simulink model "sampleModel2090"  (R2023a)
settings: Solver=VariableStepAuto  StartTime=0.0  StopTime=10.0  RelTol=1e-3
libraries: hdlsllib x8
settings Model: Creator=user1  LastModifiedBy=user1

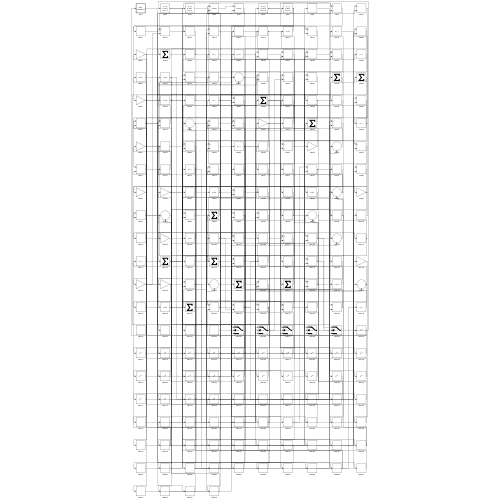
[thumbnail: Simulink's stored preview of the top-level diagram]
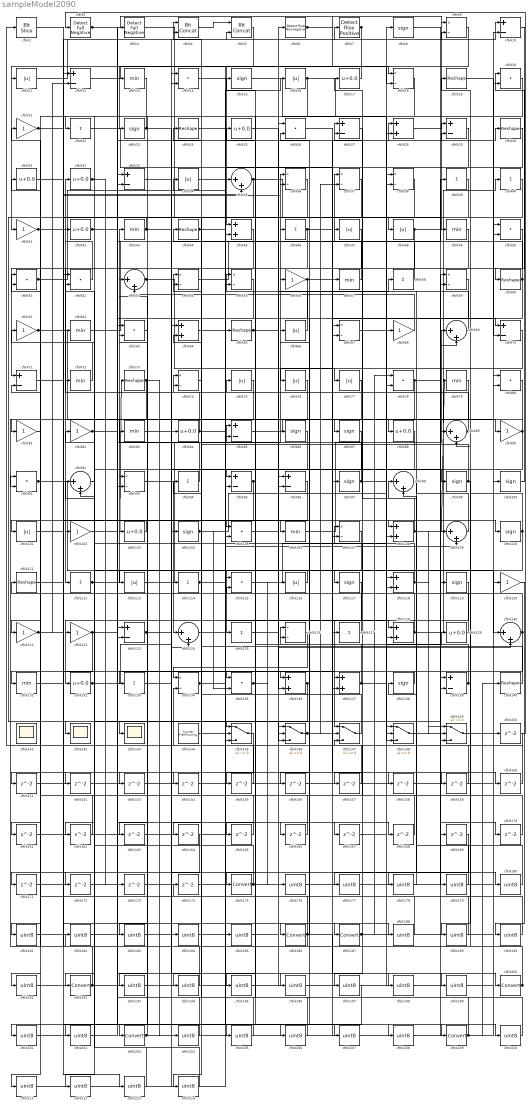
== system sampleModel2090 ==
  cfblk1 : hdlsllib/Logic and Bit Operations/Bit Slice  lidx=7  ridx=0
  cfblk{10,12,27,29,33,70..71,85,95..96,123,139} (12 alike) : Sum  Inputs=+-
  cfblk{8,15,23,86..87,97,99..100,104,110,117,119,138} (13 alike) : Signum
  cfblk{11,16,34,47..48,66,75..77,101,113,116} (12 alike) : Abs  SaturateOnIntegerOverflow=off
  cfblk{21,41,56,61,68,81..82,90,102,120..122} (12 alike) : Gain
  cfblk{17,25,31..32,42,84,88,103,129,132} (10 alike) : Bias  Bias=0.0  SaturateOnIntegerOverflow=off
  cfblk{14,20,26,50..52,63,78,80,91,105,115,135} (13 alike) : DotProduct  OutDataTypeStr=Inherit: Inherit via internal rule
  cfblk{13,43,49,57,62,72,79,83,106,131} (10 alike) : MinMax
  cfblk{9,18,36..38,54..55,59,67,74,93,107,126,134} (14 alike) : Product  Inputs=*/  RndMeth=Zero  SaturateOnIntegerOverflow=on
  cfblk{28,45,64,108,118,128,136..137} (8 alike) : Sum
  cfblk{35,53,69,89,92,98,109,124,130} (9 alike) : Sum  Inputs=|++
  cfblk{19,24,30,44,60,65,73,111,140} (9 alike) : Reshape
  cfblk{22,39..40,46,58,94,112,114,125,127,133} (11 alike) : Sum  Inputs=+
  cfblk141 : Scope
      settings: Floating=on
  cfblk142 : Scope
  cfblk143 : Scope
  cfblk144 : hdlsllib/Sources/Counter Free-Running  NumBits=16  tsamp=-1
  cfblk{145..149} (5 alike) : Switch  SaturateOnIntegerOverflow=off  InputSameDT=off
  cfblk{150..174} (25 alike) : Delay  SampleTime=1
  cfblk{175,186..187,192,200,203,209} (7 alike) : DataTypeConversion  SaturateOnIntegerOverflow=off  RndMeth=Floor
  cfblk{176..185,188..191,193..199,201..202,204..208,210..214} (33 alike) : DataTypeConversion  OutDataTypeStr=uint8  SaturateOnIntegerOverflow=off  RndMeth=Floor
  cfblk2 : hdlsllib/Logic and Bit Operations/Detect Fall Negative  vinit=0  OutDataTypeStr=boolean
  cfblk3 : hdlsllib/Logic and Bit Operations/Detect Fall Negative  vinit=0  OutDataTypeStr=boolean
  cfblk4 : hdlsllib/Logic and Bit Operations/Bit Concat  numInputs=2
  cfblk5 : hdlsllib/Logic and Bit Operations/Bit Concat  numInputs=2
  cfblk6 : hdlsllib/Logic and Bit Operations/Detect Rise Nonnegative  vinit=0  OutDataTypeStr=boolean
  cfblk7 : hdlsllib/Logic and Bit Operations/Detect Rise Positive  vinit=0  OutDataTypeStr=boolean
  wires:
  cfblk94/1 -> cfblk43/1
  cfblk86/1 -> cfblk192/1
  cfblk107/1 -> cfblk125/1
  cfblk128/1 -> cfblk40/1, cfblk54/2
  cfblk43/1 -> cfblk142/1, cfblk105/1
  cfblk52/1 -> cfblk32/1
  cfblk112/1 -> cfblk73/1, cfblk46/1, cfblk168/1
  cfblk44/1 -> cfblk166/1, cfblk167/1
  cfblk3/1 -> cfblk136/1
  cfblk2/1 -> cfblk49/1, cfblk148/3
  cfblk55/1 -> cfblk123/2
  cfblk42/1 -> cfblk3/1, cfblk137/2
  cfblk126/1 -> cfblk134/1
  cfblk45/1 -> cfblk112/1
  cfblk7/1 -> cfblk45/1, cfblk23/1
  cfblk77/1 -> cfblk103/1
  cfblk133/1 -> cfblk84/1
  cfblk57/1 -> cfblk37/1
  cfblk64/1 -> cfblk187/1
  cfblk31/1 -> cfblk106/1
  cfblk66/1 -> cfblk36/1
  cfblk18/1 -> cfblk95/1
  cfblk73/1 -> cfblk93/2, cfblk184/1
  cfblk85/1 -> cfblk90/1
  cfblk10/1 -> cfblk60/1
  cfblk28/1 -> cfblk29/1
  cfblk27/1 -> cfblk87/1
  cfblk117/1 -> cfblk147/1
  cfblk106/1 -> cfblk69/1
  cfblk122/1 -> cfblk85/1, cfblk131/1
  cfblk9/1 -> cfblk41/1
  cfblk37/1 -> cfblk81/1
  cfblk119/1 -> cfblk132/1
  cfblk90/1 -> cfblk83/1, cfblk156/1
  cfblk89/1 -> cfblk25/1, cfblk4/2
  cfblk108/1 -> cfblk79/1, cfblk17/1, cfblk149/1
  cfblk115/1 -> cfblk8/1
  cfblk65/1 -> cfblk145/1, cfblk58/1, cfblk130/2, cfblk165/1
  cfblk113/1 -> cfblk56/1
  cfblk48/1 -> cfblk119/1, cfblk205/1
  cfblk8/1 -> cfblk139/1
  cfblk4/1 -> cfblk5/1
  cfblk139/1 -> cfblk126/1, cfblk15/1
  cfblk5/1 -> cfblk85/2
  cfblk51/1 -> cfblk34/1, cfblk188/1
  cfblk33/1 -> cfblk200/1
  cfblk125/1 -> cfblk27/1
  cfblk35/1 -> cfblk69/2, cfblk191/1
  cfblk62/1 -> cfblk39/1
  cfblk22/1 -> cfblk97/1
  cfblk69/1 -> cfblk27/2
  cfblk67/1 -> cfblk68/1
  cfblk146/1 -> cfblk57/1, cfblk37/2
  cfblk47/1 -> cfblk71/1
  cfblk50/1 -> cfblk175/1
  cfblk56/1 -> cfblk70/1, cfblk30/1, cfblk133/1
  cfblk72/1 -> cfblk21/1
  cfblk88/1 -> cfblk117/1
  cfblk93/1 -> cfblk124/1
  cfblk14/1 -> cfblk209/1
  cfblk97/1 -> cfblk148/1, cfblk54/1
  cfblk135/1 -> cfblk116/1, cfblk176/1
  cfblk63/1 -> cfblk203/1
  cfblk58/1 -> cfblk44/1
  cfblk137/1 -> cfblk75/1, cfblk129/1
  cfblk24/1 -> cfblk128/1
  cfblk68/1 -> cfblk53/2
  cfblk15/1 -> cfblk78/2
  cfblk140/1 -> cfblk74/1
  cfblk21/1 -> cfblk35/2, cfblk151/1
  cfblk76/1 -> cfblk91/2
  cfblk41/1 -> cfblk28/1, cfblk36/2
  cfblk46/1 -> cfblk67/1, cfblk121/1, cfblk110/1, cfblk160/1
  cfblk34/1 -> cfblk16/1
  cfblk12/1 -> cfblk18/1
  cfblk130/1 -> cfblk107/1, cfblk153/1
  cfblk19/1 -> cfblk70/2
  cfblk53/1 -> cfblk143/1, cfblk127/1
  cfblk83/1 -> cfblk95/2
  cfblk136/1 -> cfblk162/1, cfblk163/1
  cfblk91/1 -> cfblk130/1, cfblk5/2
  cfblk138/1 -> cfblk135/1
  cfblk11/1 -> cfblk7/1
  cfblk70/1 -> cfblk76/1
  cfblk84/1 -> cfblk42/1, cfblk99/1
  cfblk74/1 -> cfblk24/1
  cfblk54/1 -> cfblk6/1
  cfblk95/1 -> cfblk154/1, cfblk155/1
  cfblk99/1 -> cfblk4/1, cfblk189/1
  cfblk32/1 -> cfblk173/1, cfblk202/1
  cfblk16/1 -> cfblk118/1, cfblk93/1
  cfblk81/1 -> cfblk51/1
  cfblk61/1 -> cfblk88/1, cfblk145/3
  cfblk102/1 -> cfblk114/1
  cfblk116/1 -> cfblk113/1
  cfblk123/1 -> cfblk180/1, cfblk204/1
  cfblk104/1 -> cfblk28/2, cfblk135/2
  cfblk149/1 -> cfblk2/1
  cfblk30/1 -> cfblk45/2
  cfblk127/1 -> cfblk31/1
  cfblk17/1 -> cfblk11/1
  cfblk40/1 -> cfblk102/1
  cfblk1/1 -> cfblk48/1
  cfblk105/1 -> cfblk137/1
  cfblk144/1 -> cfblk186/1
  cfblk82/1 -> cfblk146/3, cfblk29/2
  cfblk110/1 -> cfblk122/1, cfblk19/1
  cfblk134/1 -> cfblk74/2, cfblk149/3
  cfblk114/1 -> cfblk109/2, cfblk214/1
  cfblk109/1 -> cfblk55/1
  cfblk78/1 -> cfblk170/1, cfblk171/1
  cfblk147/1 -> cfblk94/1
  cfblk103/1 -> cfblk101/1
  cfblk118/1 -> cfblk72/1, cfblk149/2
  cfblk60/1 -> cfblk47/1, cfblk195/1
  cfblk49/1 -> cfblk67/2
  cfblk121/1 -> cfblk145/2, cfblk9/2, cfblk12/2
  cfblk6/1 -> cfblk9/1, cfblk18/2
  cfblk101/1 -> cfblk136/2
  cfblk39/1 -> cfblk148/2
  cfblk100/1 -> cfblk20/1
  cfblk129/1 -> cfblk66/1
  cfblk25/1 -> cfblk108/1
  cfblk23/1 -> cfblk22/1, cfblk124/2
  cfblk29/1 -> cfblk77/1
  cfblk132/1 -> cfblk10/1, cfblk198/1
  cfblk150/1 -> cfblk1/1
  cfblk151/1 -> cfblk146/1
  cfblk87/1 -> cfblk152/1
  cfblk153/1 -> cfblk10/2
  cfblk154/1 -> cfblk146/2
  cfblk155/1 -> cfblk134/2
  cfblk156/1 -> cfblk118/2
  cfblk79/1 -> cfblk157/1
  cfblk157/1 -> cfblk147/2
  cfblk26/1 -> cfblk158/1
  cfblk124/1 -> cfblk159/1
  cfblk159/1 -> cfblk126/2
  cfblk160/1 -> cfblk51/2
  cfblk145/1 -> cfblk161/1
  cfblk161/1 -> cfblk35/1
  cfblk162/1 -> cfblk71/2
  cfblk163/1 -> cfblk105/2
  cfblk36/1 -> cfblk164/1
  cfblk165/1 -> cfblk52/1
  cfblk166/1 -> cfblk123/1
  cfblk167/1 -> cfblk108/2
  cfblk168/1 -> cfblk147/3
  cfblk148/1 -> cfblk169/1
  cfblk170/1 -> cfblk55/2
  cfblk171/1 -> cfblk128/2
  cfblk20/1 -> cfblk172/1
  cfblk172/1 -> cfblk109/1
  cfblk173/1 -> cfblk139/2
  cfblk175/1 -> cfblk150/1, cfblk52/2
  cfblk176/1 -> cfblk50/1
  cfblk169/1 -> cfblk177/1
  cfblk177/1 -> cfblk50/2
  cfblk98/1 -> cfblk178/1
  cfblk178/1 -> cfblk138/1
  cfblk158/1 -> cfblk179/1
  cfblk179/1 -> cfblk98/1
  cfblk180/1 -> cfblk98/2
  cfblk13/1 -> cfblk181/1
  cfblk181/1 -> cfblk104/1
  cfblk182/1 -> cfblk13/1
  cfblk96/1 -> cfblk183/1
  cfblk183/1 -> cfblk26/1
  cfblk184/1 -> cfblk96/1
  cfblk185/1 -> cfblk96/2
  cfblk186/1 -> cfblk182/1, cfblk62/1, cfblk26/2, cfblk199/1
  cfblk187/1 -> cfblk100/1, cfblk78/1
  cfblk188/1 -> cfblk64/1
  cfblk189/1 -> cfblk64/2
  cfblk120/1 -> cfblk190/1
  cfblk190/1 -> cfblk61/1
  cfblk191/1 -> cfblk120/1
  cfblk192/1 -> cfblk89/1, cfblk12/1, cfblk91/1
  cfblk75/1 -> cfblk193/1
  cfblk193/1 -> cfblk86/1
  cfblk38/1 -> cfblk194/1
  cfblk194/1 -> cfblk111/1
  cfblk195/1 -> cfblk38/1
  cfblk174/1 -> cfblk196/1
  cfblk196/1 -> cfblk38/2
  cfblk80/1 -> cfblk197/1
  cfblk198/1 -> cfblk80/1
  cfblk199/1 -> cfblk80/2
  cfblk200/1 -> cfblk89/2, cfblk82/1
  cfblk164/1 -> cfblk201/1
  cfblk201/1 -> cfblk33/1
  cfblk202/1 -> cfblk33/2
  cfblk203/1 -> cfblk185/1, cfblk20/2, cfblk107/2, cfblk53/1
  cfblk204/1 -> cfblk63/1
  cfblk205/1 -> cfblk63/2
  cfblk59/1 -> cfblk206/1
  cfblk206/1 -> cfblk115/1
  cfblk71/1 -> cfblk207/1
  cfblk207/1 -> cfblk59/1
  cfblk152/1 -> cfblk208/1
  cfblk208/1 -> cfblk59/2
  cfblk209/1 -> cfblk174/1, cfblk140/1, cfblk115/2
  cfblk111/1 -> cfblk210/1
  cfblk210/1 -> cfblk14/1
  cfblk197/1 -> cfblk211/1
  cfblk211/1 -> cfblk14/2
  cfblk92/1 -> cfblk212/1
  cfblk212/1 -> cfblk65/1
  cfblk131/1 -> cfblk213/1
  cfblk213/1 -> cfblk92/1
  cfblk214/1 -> cfblk92/2
